simulink model "P3"  (R2025b)
settings: Solver=VariableStepAuto  StartTime=0.0  StopTime=30  RelTol=1e-3
undefined symbols (not defined in the file): g2r, r2g
settings Model: Creator=chenfu  LastModifiedBy=chenfu

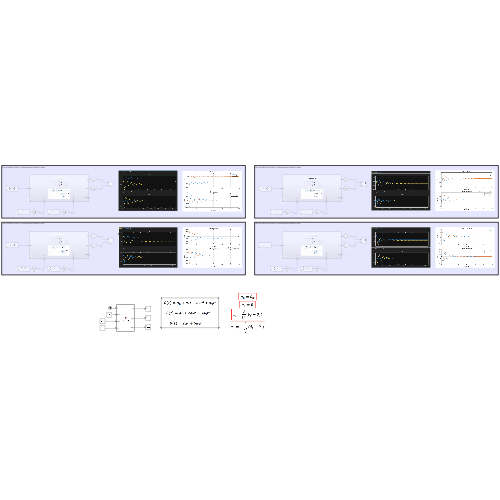
[thumbnail: Simulink's stored preview of the top-level diagram]
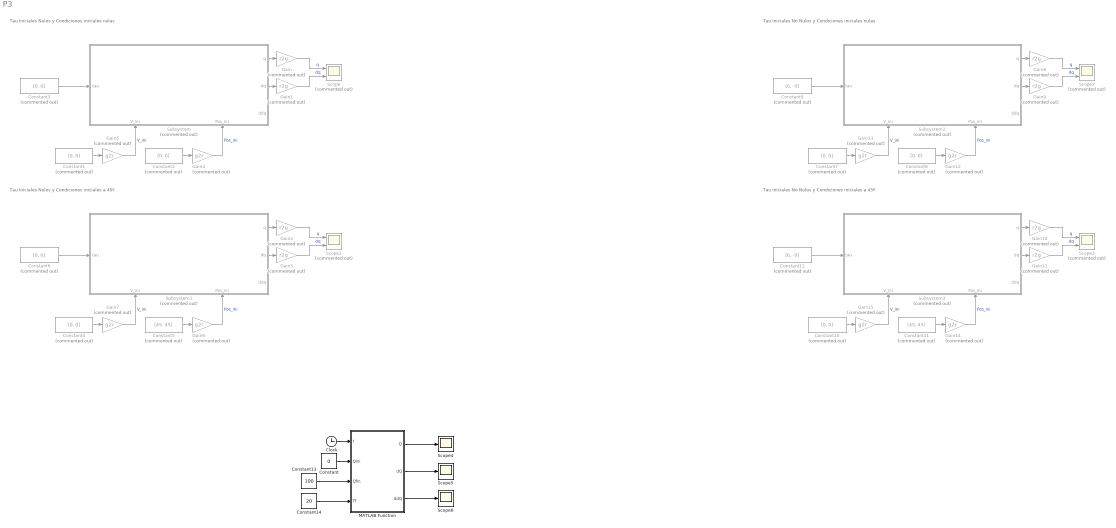
== system P3 ==
  note: Tau Iniciales Nulos y Condiciones iniciales nulas
  note: Tau Iniciales Nulos y Condiciones iniciales a 45º
  note: Tau Iniciales No Nulos y Condiciones iniciales a 45º
  note: Tau Iniciales No Nulos y Condiciones iniciales nulas
  Clock : Clock
  Constant : Constant  Value=0
  Constant{1..4,6..8,10} (8 alike) : Constant  Commented=on  Value=[0, 0]
  Constant11 : Constant  Commented=on  Value=[45, 45]
  Constant12 : Constant  Commented=on  Value=[6, -9]
  Constant13 : Constant  Value=100
  Constant14 : Constant  Value=20
  Constant5 : Constant  Commented=on  Value=[45, 45]
  Constant9 : Constant  Commented=on  Value=[6, -9]
  Gain{,1..3,8..11} (8 alike) : Gain  Commented=on  Gain=r2g
  Gain{4..7,12..15} (8 alike) : Gain  Commented=on  Gain=g2r
  MATLAB Function : MATLAB Function  TreatAsAtomicUnit=on
  Scope{,1..3} (4 alike) : Scope  Commented=on  NumInputPorts=2
      Scope settings: ActiveDisplayYMinimum=-1  ActiveDisplayYMaximum=1
      Scope1 settings: ActiveDisplayYMinimum=-196.19639795695974  ActiveDisplayYMaximum=108.3534460158745
      Scope2 settings: ActiveDisplayYMinimum=-156.87856236125987  ActiveDisplayYMaximum=17.430951373473317  DataLoggingVariableName=ScopeData2
      Scope3 settings: ActiveDisplayYMinimum=-186.99108870014706  ActiveDisplayYMaximum=70.77678763334967  DataLoggingVariableName=ScopeData3
  Scope4 : Scope
      settings: ActiveDisplayYMinimum=-12.496274999999997  ActiveDisplayYMaximum=112.466475  DataLoggingVariableName=ScopeData4
  Scope5 : Scope
      settings: ActiveDisplayYMinimum=-26.249625000000012  ActiveDisplayYMaximum=11.246625  DataLoggingVariableName=ScopeData5
  Scope6 : Scope
      settings: ActiveDisplayYMinimum=-3.5625000000000009  ActiveDisplayYMaximum=2.0625  DataLoggingVariableName=ScopeData6
  Subsystem : Subsystem  Commented=on
      settings: PortSchema="{\"entries\":[{\"content\":{\"sides\":[{\"content\":{\"connectorIds\":[\"In1\"]},\"type\":\"ConnectorPlacement.EquallySpacedRectSide\",\"uuid\":\"2e97471b-8716-4735-a3ba-83b196a16c3f\"},{\"content\":{\"connectorIds\":[\"Out1\",\"Out2\",\"Out3\"],\"side\":\"RIGHT\"},\"type\":\"ConnectorPlacement.EquallySpacedRectSide\",\"uuid\":\"0e7d6fbc-499a-459c-841f-ec0d30b56268\"},{\"content\":{\"side\":\"TOP\"},\"type\":\"ConnectorPlacement.EquallySpacedRectSide\",\"uuid\":\"4fa0b941-b86a-44a8-a051-5076c17c6f35\"},{\"content\":{\"connectorIds\":[\"In2\",\"In3\"],\"side\":\"BOTTOM\"},\"type\":\"ConnectorPlacement.EquallySpacedRectSide\",\"uuid\":\"1c6ff8a8-e8be-4b29-84c9-63cf84561027\"}]},\"type\":\"ConnectorPlacement.EquallySpacedConnector\",\"uuid\":\"8f41eaed-d9b5-45d3-9178-66754a425a67\"}],\"packageUris\":[\"http://schema.mathworks.com/mf0/Connector/R2020b\"],\"version\":\"1.0\"}"
  Subsystem1 : Subsystem  Commented=on
      settings: PortSchema="{\"entries\":[{\"content\":{\"sides\":[{\"content\":{\"connectorIds\":[\"In1\"]},\"type\":\"ConnectorPlacement.EquallySpacedRectSide\",\"uuid\":\"2e97471b-8716-4735-a3ba-83b196a16c3f\"},{\"content\":{\"connectorIds\":[\"Out1\",\"Out2\",\"Out3\"],\"side\":\"RIGHT\"},\"type\":\"ConnectorPlacement.EquallySpacedRectSide\",\"uuid\":\"0e7d6fbc-499a-459c-841f-ec0d30b56268\"},{\"content\":{\"side\":\"TOP\"},\"type\":\"ConnectorPlacement.EquallySpacedRectSide\",\"uuid\":\"4fa0b941-b86a-44a8-a051-5076c17c6f35\"},{\"content\":{\"connectorIds\":[\"In2\",\"In3\"],\"side\":\"BOTTOM\"},\"type\":\"ConnectorPlacement.EquallySpacedRectSide\",\"uuid\":\"1c6ff8a8-e8be-4b29-84c9-63cf84561027\"}]},\"type\":\"ConnectorPlacement.EquallySpacedConnector\",\"uuid\":\"8f41eaed-d9b5-45d3-9178-66754a425a67\"}],\"packageUris\":[\"http://schema.mathworks.com/mf0/Connector/R2020b\"],\"version\":\"1.0\"}"
  Subsystem2 : Subsystem  Commented=on
      settings: PortSchema="{\"entries\":[{\"content\":{\"sides\":[{\"content\":{\"connectorIds\":[\"In1\"]},\"type\":\"ConnectorPlacement.EquallySpacedRectSide\",\"uuid\":\"2e97471b-8716-4735-a3ba-83b196a16c3f\"},{\"content\":{\"connectorIds\":[\"Out1\",\"Out2\",\"Out3\"],\"side\":\"RIGHT\"},\"type\":\"ConnectorPlacement.EquallySpacedRectSide\",\"uuid\":\"0e7d6fbc-499a-459c-841f-ec0d30b56268\"},{\"content\":{\"side\":\"TOP\"},\"type\":\"ConnectorPlacement.EquallySpacedRectSide\",\"uuid\":\"4fa0b941-b86a-44a8-a051-5076c17c6f35\"},{\"content\":{\"connectorIds\":[\"In2\",\"In3\"],\"side\":\"BOTTOM\"},\"type\":\"ConnectorPlacement.EquallySpacedRectSide\",\"uuid\":\"1c6ff8a8-e8be-4b29-84c9-63cf84561027\"}]},\"type\":\"ConnectorPlacement.EquallySpacedConnector\",\"uuid\":\"8f41eaed-d9b5-45d3-9178-66754a425a67\"}],\"packageUris\":[\"http://schema.mathworks.com/mf0/Connector/R2020b\"],\"version\":\"1.0\"}"
  Subsystem3 : Subsystem  Commented=on
      settings: PortSchema="{\"entries\":[{\"content\":{\"sides\":[{\"content\":{\"connectorIds\":[\"In1\"]},\"type\":\"ConnectorPlacement.EquallySpacedRectSide\",\"uuid\":\"2e97471b-8716-4735-a3ba-83b196a16c3f\"},{\"content\":{\"connectorIds\":[\"Out1\",\"Out2\",\"Out3\"],\"side\":\"RIGHT\"},\"type\":\"ConnectorPlacement.EquallySpacedRectSide\",\"uuid\":\"0e7d6fbc-499a-459c-841f-ec0d30b56268\"},{\"content\":{\"side\":\"TOP\"},\"type\":\"ConnectorPlacement.EquallySpacedRectSide\",\"uuid\":\"4fa0b941-b86a-44a8-a051-5076c17c6f35\"},{\"content\":{\"connectorIds\":[\"In2\",\"In3\"],\"side\":\"BOTTOM\"},\"type\":\"ConnectorPlacement.EquallySpacedRectSide\",\"uuid\":\"1c6ff8a8-e8be-4b29-84c9-63cf84561027\"}]},\"type\":\"ConnectorPlacement.EquallySpacedConnector\",\"uuid\":\"8f41eaed-d9b5-45d3-9178-66754a425a67\"}],\"packageUris\":[\"http://schema.mathworks.com/mf0/Connector/R2020b\"],\"version\":\"1.0\"}"
  wires:
  Constant3/1 -> Subsystem/1(tau)
  Constant1/1 -> Gain5/1
  Constant2/1 -> Gain4/1
  Subsystem/1(q) -> Gain/1
  Subsystem/2(dq) -> Gain1/1
  Gain/1 -> Scope/1  "q"
  Gain1/1 -> Scope/2  "dq"
  Gain4/1 -> Subsystem/3(Pos_ini)  "Pos_ini"
  Gain5/1 -> Subsystem/2(V_ini)  "V_ini"
  Gain7/1 -> Subsystem1/2(V_ini)  "V_ini"
  Constant6/1 -> Subsystem1/1(tau)
  Subsystem1/2(dq) -> Gain3/1
  Constant5/1 -> Gain6/1
  Gain2/1 -> Scope1/1  "q"
  Gain3/1 -> Scope1/2  "dq"
  Subsystem1/1(q) -> Gain2/1
  Gain6/1 -> Subsystem1/3(Pos_ini)  "Pos_ini"
  Constant4/1 -> Gain7/1
  Gain9/1 -> Scope2/2  "dq"
  Gain12/1 -> Subsystem2/3(Pos_ini)  "Pos_ini"
  Subsystem3/2(dq) -> Gain11/1
  Gain8/1 -> Scope2/1  "q"
  Subsystem2/1(q) -> Gain8/1
  Constant8/1 -> Gain12/1
  Gain15/1 -> Subsystem3/2(V_ini)  "V_ini"
  Subsystem2/2(dq) -> Gain9/1
  Constant9/1 -> Subsystem2/1(tau)
  Subsystem3/1(q) -> Gain10/1
  Gain14/1 -> Subsystem3/3(Pos_ini)  "Pos_ini"
  Gain10/1 -> Scope3/1  "q"
  Constant10/1 -> Gain15/1
  Gain11/1 -> Scope3/2  "dq"
  Gain13/1 -> Subsystem2/2(V_ini)  "V_ini"
  Constant12/1 -> Subsystem3/1(tau)
  Constant11/1 -> Gain14/1
  Constant7/1 -> Gain13/1
  Constant/1 -> MATLAB Function/2(Qini)
  Constant13/1 -> MATLAB Function/3(Qfin)
  Constant14/1 -> MATLAB Function/4(Tf)
  Clock/1 -> MATLAB Function/1(t)
  MATLAB Function/1(Q) -> Scope4/1
  MATLAB Function/2(dQ) -> Scope5/1
  MATLAB Function/3(ddQ) -> Scope6/1

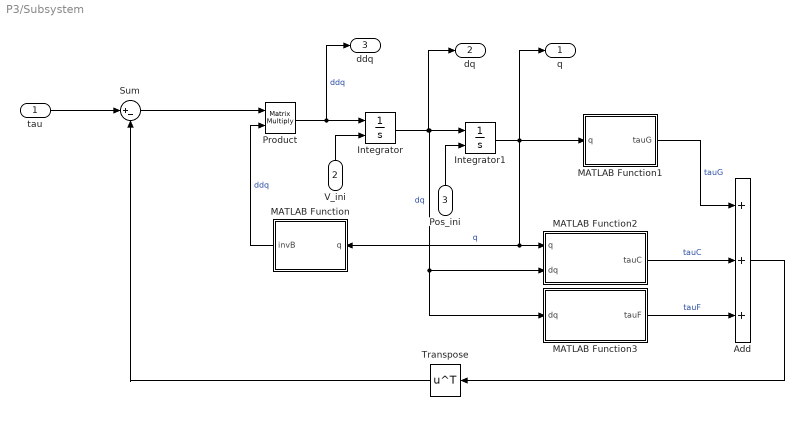
== system P3/Subsystem ==
  tau : Inport
  V_ini : Inport  Port=2
  Pos_ini : Inport  Port=3
  Add : Sum  Inputs=+++
  Integrator : Integrator  InitialConditionSource=external
  Integrator1 : Integrator  InitialConditionSource=external
  MATLAB Function : MATLAB Function  TreatAsAtomicUnit=on
  MATLAB Function1 : MATLAB Function  TreatAsAtomicUnit=on
  MATLAB Function2 : MATLAB Function  TreatAsAtomicUnit=on
  MATLAB Function3 : MATLAB Function  TreatAsAtomicUnit=on
  Product : Product  Multiplication=Matrix(*)
  Sum : Sum  Inputs=|+-
  Transpose : Math  Operator=transpose
  q : Outport
  dq : Outport  Port=2
  ddq : Outport  Port=3
  wires:
  MATLAB Function2/1(tauC) -> Add/2  "tauC"
  tau/1 -> Sum/1
  V_ini/1 -> Integrator/2
  MATLAB Function/1(invB) -> Product/2  "ddq"
  Add/1 -> Transpose/1
  MATLAB Function1/1(tauG) -> Add/1  "tauG"
  Sum/1 -> Product/1
  Integrator/1 -> dq/1, Integrator1/1, MATLAB Function3/1(dq), MATLAB Function2/2(dq)  "dq"
  Pos_ini/1 -> Integrator1/2
  Product/1 -> ddq/1, Integrator/1  "ddq"
  MATLAB Function3/1(tauF) -> Add/3  "tauF"
  Integrator1/1 -> q/1, MATLAB Function1/1(q), MATLAB Function/1(q), MATLAB Function2/1(q)  "q"
  Transpose/1 -> Sum/2

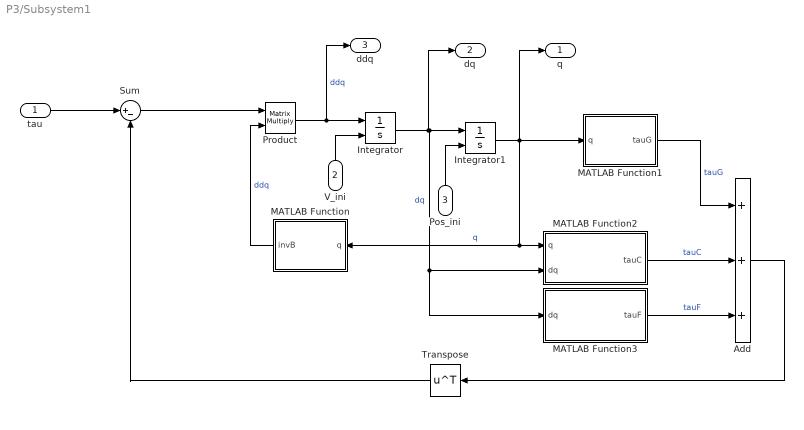
== system P3/Subsystem1 ==
  tau : Inport
  V_ini : Inport  Port=2
  Pos_ini : Inport  Port=3
  Add : Sum  Inputs=+++
  Integrator : Integrator  InitialConditionSource=external
  Integrator1 : Integrator  InitialConditionSource=external
  MATLAB Function : MATLAB Function  TreatAsAtomicUnit=on
  MATLAB Function1 : MATLAB Function  TreatAsAtomicUnit=on
  MATLAB Function2 : MATLAB Function  TreatAsAtomicUnit=on
  MATLAB Function3 : MATLAB Function  TreatAsAtomicUnit=on
  Product : Product  Multiplication=Matrix(*)
  Sum : Sum  Inputs=|+-
  Transpose : Math  Operator=transpose
  q : Outport
  dq : Outport  Port=2
  ddq : Outport  Port=3
  wires:
  MATLAB Function2/1(tauC) -> Add/2  "tauC"
  tau/1 -> Sum/1
  V_ini/1 -> Integrator/2
  MATLAB Function/1(invB) -> Product/2  "ddq"
  Add/1 -> Transpose/1
  MATLAB Function1/1(tauG) -> Add/1  "tauG"
  Sum/1 -> Product/1
  Integrator/1 -> dq/1, Integrator1/1, MATLAB Function3/1(dq), MATLAB Function2/2(dq)  "dq"
  Pos_ini/1 -> Integrator1/2
  Product/1 -> ddq/1, Integrator/1  "ddq"
  MATLAB Function3/1(tauF) -> Add/3  "tauF"
  Integrator1/1 -> q/1, MATLAB Function1/1(q), MATLAB Function/1(q), MATLAB Function2/1(q)  "q"
  Transpose/1 -> Sum/2

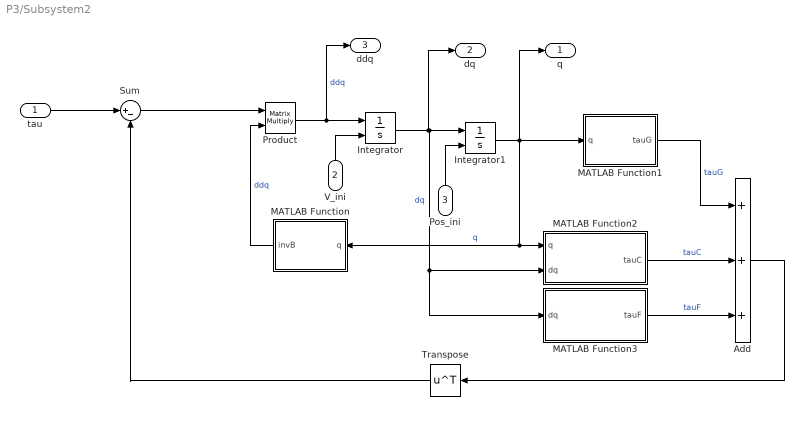
== system P3/Subsystem2 ==
  tau : Inport
  V_ini : Inport  Port=2
  Pos_ini : Inport  Port=3
  Add : Sum  Inputs=+++
  Integrator : Integrator  InitialConditionSource=external
  Integrator1 : Integrator  InitialConditionSource=external
  MATLAB Function : MATLAB Function  TreatAsAtomicUnit=on
  MATLAB Function1 : MATLAB Function  TreatAsAtomicUnit=on
  MATLAB Function2 : MATLAB Function  TreatAsAtomicUnit=on
  MATLAB Function3 : MATLAB Function  TreatAsAtomicUnit=on
  Product : Product  Multiplication=Matrix(*)
  Sum : Sum  Inputs=|+-
  Transpose : Math  Operator=transpose
  q : Outport
  dq : Outport  Port=2
  ddq : Outport  Port=3
  wires:
  MATLAB Function2/1(tauC) -> Add/2  "tauC"
  tau/1 -> Sum/1
  V_ini/1 -> Integrator/2
  MATLAB Function/1(invB) -> Product/2  "ddq"
  Add/1 -> Transpose/1
  MATLAB Function1/1(tauG) -> Add/1  "tauG"
  Sum/1 -> Product/1
  Integrator/1 -> dq/1, Integrator1/1, MATLAB Function3/1(dq), MATLAB Function2/2(dq)  "dq"
  Pos_ini/1 -> Integrator1/2
  Product/1 -> ddq/1, Integrator/1  "ddq"
  MATLAB Function3/1(tauF) -> Add/3  "tauF"
  Integrator1/1 -> q/1, MATLAB Function1/1(q), MATLAB Function/1(q), MATLAB Function2/1(q)  "q"
  Transpose/1 -> Sum/2

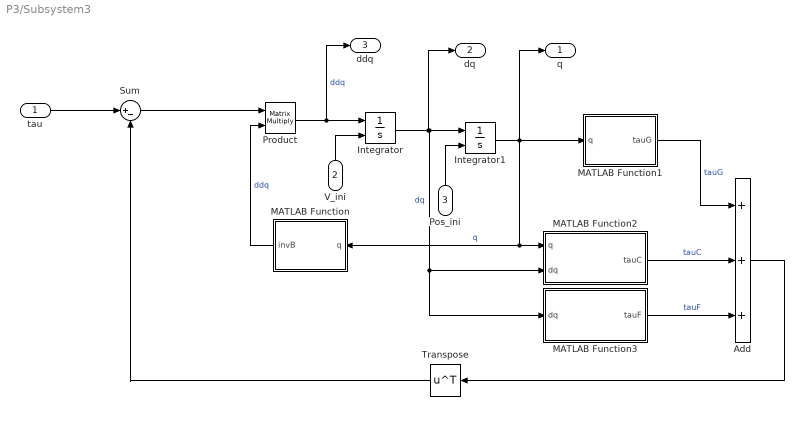
== system P3/Subsystem3 ==
  tau : Inport
  V_ini : Inport  Port=2
  Pos_ini : Inport  Port=3
  Add : Sum  Inputs=+++
  Integrator : Integrator  InitialConditionSource=external
  Integrator1 : Integrator  InitialConditionSource=external
  MATLAB Function : MATLAB Function  TreatAsAtomicUnit=on
  MATLAB Function1 : MATLAB Function  TreatAsAtomicUnit=on
  MATLAB Function2 : MATLAB Function  TreatAsAtomicUnit=on
  MATLAB Function3 : MATLAB Function  TreatAsAtomicUnit=on
  Product : Product  Multiplication=Matrix(*)
  Sum : Sum  Inputs=|+-
  Transpose : Math  Operator=transpose
  q : Outport
  dq : Outport  Port=2
  ddq : Outport  Port=3
  wires:
  MATLAB Function2/1(tauC) -> Add/2  "tauC"
  tau/1 -> Sum/1
  V_ini/1 -> Integrator/2
  MATLAB Function/1(invB) -> Product/2  "ddq"
  Add/1 -> Transpose/1
  MATLAB Function1/1(tauG) -> Add/1  "tauG"
  Sum/1 -> Product/1
  Integrator/1 -> dq/1, Integrator1/1, MATLAB Function3/1(dq), MATLAB Function2/2(dq)  "dq"
  Pos_ini/1 -> Integrator1/2
  Product/1 -> ddq/1, Integrator/1  "ddq"
  MATLAB Function3/1(tauF) -> Add/3  "tauF"
  Integrator1/1 -> q/1, MATLAB Function1/1(q), MATLAB Function/1(q), MATLAB Function2/1(q)  "q"
  Transpose/1 -> Sum/2

== matlab function P3/Subsystem3/MATLAB Function ==
  data: invB output; q input
function invB = Calculo_invB(q)

% Entradas
c2 = cos(q(2));

% Parámetros
m1 = 5;
m2 = 2;
L1 = 1;  
L2 = 0.6;



% B(q)
B = [
        m1*L1^2 + m2*L1^2 + 2*m2*L1*L2*c2 + m2*L2^2  ,  m2*L2^2 + m2*L2*L1*c2 ;
        m2*L2^2 + m2*L2*L1*c2                        ,  m2*L2^2            
    ];

invB = inv(B);

== matlab function P3/Subsystem3/MATLAB Function1 ==
  data: tauG output; q input
function tauG = Calculo_tauG(q)

% Entradas
c1 = cos(q(1));
c12 = cos(q(1)+q(2));

% Parámetros
m1 = 5;
m2 = 2;
L1 = 1;  
L2 = 0.6;
g  = 9.8;

% G(q)
tauG =  [ 
            (m1*c1*L1 + m2*c12*L2 + m2*c1*L1)*g;
            (m2*c12*L2)*g 
        ];

== matlab function P3/Subsystem3/MATLAB Function2 ==
  data: tauC output; q input; dq input
function tauC = Calculo_tauG(q,dq)

% Entradas
dq1 = dq(1);
dq2 = dq(2);

s2 = sin(q(2));


% Parámetros
m2 = 2;
L1 = 1;  
L2 = 0.6;

% C(q,dq)*dq
tauC =  [ 
            -m2*L2*L1*s2*(2*dq1 + dq2)*dq2;
            dq1^2*m2*L2*L1*s2
        ];

== matlab function P3/Subsystem3/MATLAB Function3 ==
  data: tauF output; dq input
function tauF = Calculo_tauF(dq)

% Entradas
dq1 = dq(1);
dq2 = dq(2);

% Parámetros
Fv = [4.5 0; 0 3.5];

% Fv*dq
tauF = Fv * [dq1; dq2];

== matlab function P3/MATLAB Function ==
  data: t input; Q output; dQ output; ddQ output; Qini input; Qfin input; Tf input
function [Q, dQ, ddQ] = gen_tray(t, Qini, Qfin, Tf)


a0 = Qini;
a1 = 0;
a2 = 3/Tf^2 * (Qfin - Qini);
a3 = -2/Tf^3 * (Qfin - Qini);

Q = a0 + a1*t + a2*t^2 + a3*t^3;
dQ = a1 + 2*a2*t + 3*a3*t^2;
ddQ = 2*a2 + 6*a3*t;

== matlab function P3/Subsystem/MATLAB Function1 ==
  data: tauG output; q input
function tauG = Calculo_tauG(q)

% Entradas
c1 = cos(q(1));
c12 = cos(q(1)+q(2));

% Parámetros
m1 = 5;
m2 = 2;
L1 = 1;  
L2 = 0.6;
g  = 9.8;

% G(q)
tauG =  [ 
            (m1*c1*L1 + m2*c12*L2 + m2*c1*L1)*g;
            (m2*c12*L2)*g 
        ];

== matlab function P3/Subsystem/MATLAB Function ==
  data: invB output; q input
function invB = Calculo_invB(q)

% Entradas
c2 = cos(q(2));

% Parámetros
m1 = 5;
m2 = 2;
L1 = 1;  
L2 = 0.6;



% B(q)
B = [
        m1*L1^2 + m2*L1^2 + 2*m2*L1*L2*c2 + m2*L2^2  ,  m2*L2^2 + m2*L2*L1*c2 ;
        m2*L2^2 + m2*L2*L1*c2                        ,  m2*L2^2            
    ];

invB = inv(B);

== matlab function P3/Subsystem/MATLAB Function2 ==
  data: tauC output; q input; dq input
function tauC = Calculo_tauG(q,dq)

% Entradas
dq1 = dq(1);
dq2 = dq(2);

s2 = sin(q(2));


% Parámetros
m2 = 2;
L1 = 1;  
L2 = 0.6;

% C(q,dq)*dq
tauC =  [ 
            -m2*L2*L1*s2*(2*dq1 + dq2)*dq2;
            dq1^2*m2*L2*L1*s2
        ];

== matlab function P3/Subsystem/MATLAB Function3 ==
  data: tauF output; dq input
function tauF = Calculo_tauF(dq)

% Entradas
dq1 = dq(1);
dq2 = dq(2);

% Parámetros
Fv = [4.5 0; 0 3.5];

% Fv*dq
tauF = Fv * [dq1; dq2];

== matlab function P3/Subsystem1/MATLAB Function ==
  data: invB output; q input
function invB = Calculo_invB(q)

% Entradas
c2 = cos(q(2));

% Parámetros
m1 = 5;
m2 = 2;
L1 = 1;  
L2 = 0.6;



% B(q)
B = [
        m1*L1^2 + m2*L1^2 + 2*m2*L1*L2*c2 + m2*L2^2  ,  m2*L2^2 + m2*L2*L1*c2 ;
        m2*L2^2 + m2*L2*L1*c2                        ,  m2*L2^2            
    ];

invB = inv(B);

== matlab function P3/Subsystem1/MATLAB Function1 ==
  data: tauG output; q input
function tauG = Calculo_tauG(q)

% Entradas
c1 = cos(q(1));
c12 = cos(q(1)+q(2));

% Parámetros
m1 = 5;
m2 = 2;
L1 = 1;  
L2 = 0.6;
g  = 9.8;

% G(q)
tauG =  [ 
            (m1*c1*L1 + m2*c12*L2 + m2*c1*L1)*g;
            (m2*c12*L2)*g 
        ];

== matlab function P3/Subsystem1/MATLAB Function2 ==
  data: tauC output; q input; dq input
function tauC = Calculo_tauG(q,dq)

% Entradas
dq1 = dq(1);
dq2 = dq(2);

s2 = sin(q(2));


% Parámetros
m2 = 2;
L1 = 1;  
L2 = 0.6;

% C(q,dq)*dq
tauC =  [ 
            -m2*L2*L1*s2*(2*dq1 + dq2)*dq2;
            dq1^2*m2*L2*L1*s2
        ];

== matlab function P3/Subsystem1/MATLAB Function3 ==
  data: tauF output; dq input
function tauF = Calculo_tauF(dq)

% Entradas
dq1 = dq(1);
dq2 = dq(2);

% Parámetros
Fv = [4.5 0; 0 3.5];

% Fv*dq
tauF = Fv * [dq1; dq2];

== matlab function P3/Subsystem2/MATLAB Function ==
  data: invB output; q input
function invB = Calculo_invB(q)

% Entradas
c2 = cos(q(2));

% Parámetros
m1 = 5;
m2 = 2;
L1 = 1;  
L2 = 0.6;



% B(q)
B = [
        m1*L1^2 + m2*L1^2 + 2*m2*L1*L2*c2 + m2*L2^2  ,  m2*L2^2 + m2*L2*L1*c2 ;
        m2*L2^2 + m2*L2*L1*c2                        ,  m2*L2^2            
    ];

invB = inv(B);

== matlab function P3/Subsystem2/MATLAB Function1 ==
  data: tauG output; q input
function tauG = Calculo_tauG(q)

% Entradas
c1 = cos(q(1));
c12 = cos(q(1)+q(2));

% Parámetros
m1 = 5;
m2 = 2;
L1 = 1;  
L2 = 0.6;
g  = 9.8;

% G(q)
tauG =  [ 
            (m1*c1*L1 + m2*c12*L2 + m2*c1*L1)*g;
            (m2*c12*L2)*g 
        ];

== matlab function P3/Subsystem2/MATLAB Function2 ==
  data: tauC output; q input; dq input
function tauC = Calculo_tauG(q,dq)

% Entradas
dq1 = dq(1);
dq2 = dq(2);

s2 = sin(q(2));


% Parámetros
m2 = 2;
L1 = 1;  
L2 = 0.6;

% C(q,dq)*dq
tauC =  [ 
            -m2*L2*L1*s2*(2*dq1 + dq2)*dq2;
            dq1^2*m2*L2*L1*s2
        ];

== matlab function P3/Subsystem2/MATLAB Function3 ==
  data: tauF output; dq input
function tauF = Calculo_tauF(dq)

% Entradas
dq1 = dq(1);
dq2 = dq(2);

% Parámetros
Fv = [4.5 0; 0 3.5];

% Fv*dq
tauF = Fv * [dq1; dq2];
